simulink model "benchmark_ivan_PIANN"  (R2024b)
settings: Solver=FixedStepAuto  StartTime=0.0  StopTime=14  FixedStep=0.0001  RelTol=1e-5  AbsTol=1e-8  EnableMultiTasking=on
values from neighbouring files (symbols this model uses):
  b1 = csvread('./DAE_ANN/ANN/Biases/30_04_21/lstm_ann_pi_standard_fix_noSo4_rnn_1__100_16_b_3.csv')    [init_PI_ann.m]    (also in init_PI_ann_hier.m = csvread('./DAE_ANN/ANN/Biases/12_05_21/lstm_ann_pi_standard_; init_PI_ann_hier_v2.m = csvread('./DAE_ANN/ANN/Biases/12_05_21/lstm_ann_pi_standard_; init_PI_ann_lab.m = csvread('./DAE_ANN/ANN/Biases/12_05_21/lstm_ann_pi_standard_)
  b2 = csvread('./DAE_ANN/ANN/Biases/30_04_21/lstm_ann_pi_standard_fix_noSo4_rnn_1__100_16_b_3.csv')    [init_PI_ann.m]    (also in init_PI_ann_hier.m = csvread('./DAE_ANN/ANN/Biases/12_05_21/lstm_ann_pi_standard_; init_PI_ann_hier_v2.m = csvread('./DAE_ANN/ANN/Biases/12_05_21/lstm_ann_pi_standard_; init_PI_ann_lab.m = csvread('./DAE_ANN/ANN/Biases/12_05_21/lstm_ann_pi_standard_)
  b_last = csvread('./DAE_ANN/ANN/Biases/12_05_21/lstm_ann_pi_standard_fix_noSo4_last__100_1_b_2.csv')'    [init_PI_ann_hier.m]    (also in init_PI_ann_hier_v2.m; init_PI_ann_lab.m)
  b_out = csvread('./DAE_ANN/ANN/Biases/30_04_21/lstm_ann_pi_standard_fix_noSo4_final__100_16_b_3.csv')    [init_PI_ann.m]    (also in init_PI_ann_hier.m = csvread('./DAE_ANN/ANN/Biases/12_05_21/lstm_ann_pi_standard_; init_PI_ann_hier_v2.m = csvread('./DAE_ANN/ANN/Biases/12_05_21/lstm_ann_pi_standard_; init_PI_ann_lab.m = csvread('./DAE_ANN/ANN/Biases/12_05_21/lstm_ann_pi_standard_)
  ic_sw_Kla = 145*ones(n_sw,1)    [init_PI_ann.m]    (also in init_PI_ann_hier.m; init_PI_ann_hier_v2.m; init_PI_ann_lab.m)
  ic_sw_Snh4 = 6*ones(n_sw,1)    [init_PI_ann.m]    (also in init_PI_ann_hier.m; init_PI_ann_hier_v2.m; init_PI_ann_lab.m)
  ic_sw_Sno4 = 8*ones(n_sw,1)    [init_PI_ann.m]    (also in init_PI_ann_hier.m; init_PI_ann_hier_v2.m; init_PI_ann_lab.m)
  ic_sw_So4 = 3*ones(n_sw,1)    [init_PI_ann.m]    (also in init_PI_ann_hier.m; init_PI_ann_hier_v2.m; init_PI_ann_lab.m)
  ic_sw_So5 = 2*ones(n_sw,1)    [init_PI_ann.m]    (also in init_PI_ann_hier.m; init_PI_ann_hier_v2.m; init_PI_ann_lab.m)
  KLa5_max = 360    [sensorinit.m]
  max_Q4 = 100000    [sensorinit.m]
  max_SNH4 = 20    [sensorinit.m]
  max_SNO2 = 20    [sensorinit.m]
  max_SNO4 = 20    [sensorinit.m]
  max_SO4 = 10    [sensorinit.m]
  max_SO5 = 10    [sensorinit.m]    (also in setup_Prac5.m = 5)
  max_TSS4 = 10000    [sensorinit.m]
  mean_scaler_dir = csvread('./DAE_ANN/ANN/Scalers/30_04_21_lstm_ann_pi_standard_fix_noSo4/mean_scaler_lstm_ann_pi_standard_fix_noSo4.csv')    [init_PI_ann.m]    (also in init_PI_ann_hier.m = csvread('./DAE_ANN/ANN/Scalers/12_05_21_lstm_ann_pi_standard; init_PI_ann_hier_v2.m = csvread('./DAE_ANN/ANN/Scalers/12_05_21_lstm_ann_pi_standard; setup_Prac5.m = [(Q/k)^2, 1.9756, 0.0000, 0]')
  mean_scaler_dir_out = csvread('./DAE_ANN/ANN/Scalers/30_04_21_lstm_ann_pi_standard_fix_noSo4/mean_scaler_lstm_ann_pi_standard_fix_noSo4_out.csv')    [init_PI_ann.m]    (also in init_PI_ann_hier.m = csvread('./DAE_ANN/ANN/Scalers/12_05_21_lstm_ann_pi_standard; init_PI_ann_hier_v2.m = csvread('./DAE_ANN/ANN/Scalers/12_05_21_lstm_ann_pi_standard; setup_Prac5.m = 0)
  min_Q4 = 0    [sensorinit.m]
  min_SNH4 = 0    [sensorinit.m]
  min_SNO2 = 0    [sensorinit.m]
  min_SNO4 = 0    [sensorinit.m]
  min_SO5 = 0    [sensorinit.m]
  min_TSS4 = 0    [sensorinit.m]
  n_layers = 1    [init_PI_ann.m]    (also in init_PI_ann_hier.m; init_PI_ann_hier_v2.m; init_PI_ann_lab.m)
  n_sw = 16    [init_PI_ann.m]    (also in init_PI_ann_hier.m = 1; init_PI_ann_hier_v2.m = 1; init_PI_ann_lab.m = 1)
  n_sw_inverse = 16    [init_PI_ann.m]    (also in init_PI_ann_hier.m = 1; init_PI_ann_hier_v2.m = 1; init_PI_ann_lab.m = 1)
  noiseseed_Q4 = 1    [sensorinit.m]
  noiseseed_SNH4 = 2    [sensorinit.m]
  noiseseed_SNO2 = 2    [sensorinit.m]
  noiseseed_SNO4 = 2    [sensorinit.m]
  noiseseed_SO4 = 2    [sensorinit.m]
  noiseseed_SO5 = 1    [sensorinit.m]
  noiseseed_TSS4 = 1    [sensorinit.m]
  noisesource_Q4 = 1    [sensorinit.m]
  noisesource_SNH4 = 1    [sensorinit.m]
  noisesource_SNO2 = 1    [sensorinit.m]
  noisesource_SNO4 = 1    [sensorinit.m]
  noisesource_SO4 = 1    [sensorinit.m]
  noisesource_SO5 = 1    [sensorinit.m]
  noisesource_TSS4 = 1    [sensorinit.m]
  Qin0 = 18446    [states.mat]
  Qintr = 12141.8126939    [states.mat]
  Qintr_max = 5*Qin0    [sensorinit.m]
  Qintrawstate = 114243.527362    [states.mat]
  Qintrintstate = -116205.765277    [states.mat]
  SETTLERINIT = [12.5979803087 18.2981709885 29.6744598765 68.7829340492 352.293497132 353.981663079 351.499035887 351.323930185 355.679725774 6417.21684783 30 30 ... (80 elements, 1x80)]    [states.mat]
  Sno_mean = 1    [run_bsm1_PIANN_variable.m]
  SO5awstate = 469.399689831    [states.mat]
  SO5intstate = -450.70071346    [states.mat]
  SO5ref = 2    [run_bsm1_PIANN.m]    (also in run_bsm1_PIANN_variable.m)
  So_mean = 2    [run_bsm1_PIANN_variable.m]    (also in setup_Prac5.m = 0.2)
  std_Q4 = 0.025    [sensorinit.m]
  std_scaler_dir = csvread('./DAE_ANN/ANN/Scalers/30_04_21_lstm_ann_pi_standard_fix_noSo4/std_scaler_lstm_ann_pi_standard_fix_noSo4.csv')    [init_PI_ann.m]    (also in init_PI_ann_hier.m = csvread('./DAE_ANN/ANN/Scalers/12_05_21_lstm_ann_pi_standard; init_PI_ann_hier_v2.m = csvread('./DAE_ANN/ANN/Scalers/12_05_21_lstm_ann_pi_standard; setup_Prac5.m = [1, 0.7579, 0.05, 1]')
  std_scaler_dir_out = csvread('./DAE_ANN/ANN/Scalers/30_04_21_lstm_ann_pi_standard_fix_noSo4/std_scaler_lstm_ann_pi_standard_fix_noSo4_out.csv')    [init_PI_ann.m]    (also in init_PI_ann_hier.m = csvread('./DAE_ANN/ANN/Scalers/12_05_21_lstm_ann_pi_standard; init_PI_ann_hier_v2.m = csvread('./DAE_ANN/ANN/Scalers/12_05_21_lstm_ann_pi_standard; setup_Prac5.m = 1)
  std_SNH4 = 0.025    [sensorinit.m]
  std_SNO2 = 0.025    [sensorinit.m]
  std_SO4 = 0.025    [sensorinit.m]
  std_SO5 = 0.025    [sensorinit.m]
  std_TSS4 = 0.025    [sensorinit.m]
  T = 6.5201    [setup_Prac5.m]
  t_init = 7e-3    (= 0.007)    [run_bsm1.m]    (also in run_bsm1_PIANN_variable.m = 0.05)
  T_KLa5 = T90_KLa5/(24*60)/3.89    (= 0.000714081690945)    [sensorinit.m]
  T_Q4 = T90_Q4/(24*60)/3.89    (= 0.000178520422736)    [sensorinit.m]
  t_simulink = 1/96    (= 0.0104166666667)    [run_bsm1.m]    (also in run_bsm1_PIANN.m = -1; run_bsm1_PIANN_variable.m = 0; setup_Prac5.m = 0)
  T_SNH4 = T90_SNH4/(24*60)/11.7724    (= 0.000589891988417)    [sensorinit.m]
  T_SNO2 = T90_SNO2/(24*60)/11.7724    (= 0.000589891988417)    [sensorinit.m]
  T_SNO4 = T90_SNO4/(24*60)/11.7724    (= 0.000589891988417)    [sensorinit.m]
  T_SO5 = T90_SO5/(24*60)/3.89    (= 0.000178520422736)    [sensorinit.m]
  T_TSS4 = T90_TSS4/(24*60)/3.89    (= 0.000178520422736)    [sensorinit.m]
  t_zero_order = -1    [run_bsm1_PIANN.m]    (also in run_bsm1_PIANN_variable.m)
  u1 = csvread('./DAE_ANN/ANN/Weights/30_04_21/lstm_ann_pi_standard_fix_noSo4_rnn_1__100_16_U_3.csv')    [init_PI_ann.m]    (also in init_PI_ann_hier.m = csvread('./DAE_ANN/ANN/Weights/12_05_21/lstm_ann_pi_standard; init_PI_ann_hier_v2.m = csvread('./DAE_ANN/ANN/Weights/12_05_21/lstm_ann_pi_standard)
  u2 = csvread('./DAE_ANN/ANN/Weights/30_04_21/lstm_ann_pi_standard_fix_noSo4_rnn_1__100_16_U_3.csv')    [init_PI_ann.m]    (also in init_PI_ann_hier.m = csvread('./DAE_ANN/ANN/Weights/12_05_21/lstm_ann_pi_standard; init_PI_ann_hier_v2.m = csvread('./DAE_ANN/ANN/Weights/12_05_21/lstm_ann_pi_standard)
  useideal_KLa5 = 0    [run_bsm1.m]    (also in run_bsm1_PIANN.m = 1; run_bsm1_PIANN_variable.m = 1; sensorinit.m)
  useideal_Q4 = 1    [run_bsm1_PIANN.m]    (also in run_bsm1_PIANN_variable.m; sensorinit.m = 0)
  useideal_SNH4 = 0    [run_bsm1.m]    (also in run_bsm1_PIANN.m = 1; run_bsm1_PIANN_variable.m = 1; sensorinit.m)
  useideal_SNO2 = 1    [run_bsm1_PIANN.m]    (also in run_bsm1_PIANN_variable.m; sensorinit.m = 0)
  useideal_SNO4 = 0    [run_bsm1.m]    (also in run_bsm1_PIANN.m = 1; run_bsm1_PIANN_variable.m = 1; sensorinit.m)
  useideal_SO4 = 0    [run_bsm1.m]    (also in run_bsm1_PIANN.m = 1; run_bsm1_PIANN_variable.m = 1; sensorinit.m)
  useideal_SO5 = 0    [run_bsm1.m]    (also in run_bsm1_PIANN.m = 1; run_bsm1_PIANN_variable.m = 1; sensorinit.m)
  useideal_TSS4 = 1    [run_bsm1_PIANN.m]    (also in run_bsm1_PIANN_variable.m; sensorinit.m = 0)
  usenoise_Q4 = 0    [run_bsm1_PIANN.m]    (also in run_bsm1_PIANN_variable.m; sensorinit.m = 1)
  usenoise_SNH4 = 1    [run_bsm1.m]    (also in run_bsm1_PIANN.m = 0; run_bsm1_PIANN_variable.m = 0; sensorinit.m)
  usenoise_SNO2 = 0    [run_bsm1_PIANN.m]    (also in run_bsm1_PIANN_variable.m; sensorinit.m = 1)
  usenoise_SNO4 = 1    [run_bsm1.m]    (also in run_bsm1_PIANN.m = 0; run_bsm1_PIANN_variable.m = 0; sensorinit.m)
  usenoise_SO4 = 1    [run_bsm1.m]    (also in run_bsm1_PIANN.m = 0; run_bsm1_PIANN_variable.m = 0; sensorinit.m)
  usenoise_SO5 = 1    [run_bsm1.m]    (also in run_bsm1_PIANN.m = 0; run_bsm1_PIANN_variable.m = 0; sensorinit.m)
  usenoise_TSS4 = 0    [run_bsm1_PIANN.m]    (also in run_bsm1_PIANN_variable.m; sensorinit.m = 1)
  w1 = csvread('./DAE_ANN/ANN/Weights/30_04_21/lstm_ann_pi_standard_fix_noSo4_rnn_1__100_16_W_3.csv')    [init_PI_ann.m]    (also in init_PI_ann_hier.m = csvread('./DAE_ANN/ANN/Weights/12_05_21/lstm_ann_pi_standard; init_PI_ann_hier_v2.m = csvread('./DAE_ANN/ANN/Weights/12_05_21/lstm_ann_pi_standard; init_PI_ann_lab.m = csvread('./DAE_ANN/ANN/Weights/12_05_21/lstm_ann_pi_standard)
  w2 = csvread('./DAE_ANN/ANN/Weights/30_04_21/lstm_ann_pi_standard_fix_noSo4_rnn_1__100_16_W_3.csv')    [init_PI_ann.m]    (also in init_PI_ann_hier.m = csvread('./DAE_ANN/ANN/Weights/12_05_21/lstm_ann_pi_standard; init_PI_ann_hier_v2.m = csvread('./DAE_ANN/ANN/Weights/12_05_21/lstm_ann_pi_standard; init_PI_ann_lab.m = csvread('./DAE_ANN/ANN/Weights/12_05_21/lstm_ann_pi_standard)
  w_last = csvread('./DAE_ANN/ANN/Weights/12_05_21/lstm_ann_pi_standard_fix_noSo4_last__100_1_W_2.csv')    [init_PI_ann_hier.m]    (also in init_PI_ann_hier_v2.m; init_PI_ann_lab.m)
  w_out = csvread('./DAE_ANN/ANN/Weights/30_04_21/lstm_ann_pi_standard_fix_noSo4_final__100_16_W_3.csv')    [init_PI_ann.m]    (also in init_PI_ann_hier.m = csvread('./DAE_ANN/ANN/Weights/12_05_21/lstm_ann_pi_standard; init_PI_ann_hier_v2.m = csvread('./DAE_ANN/ANN/Weights/12_05_21/lstm_ann_pi_standard; init_PI_ann_lab.m = csvread('./DAE_ANN/ANN/Weights/12_05_21/lstm_ann_pi_standard)
  XINIT1 = [30 3.2250440682 1132.84750814 98.0848162551 2520.32093658 147.34360098 454.498440184 0.006943357113 3.54207658602 12.0720627837 1.35151294762 6.05742445882 ... (15 elements, 1x15)]    [states.mat]
  XINIT2 = [30 1.63865407136 1124.24951453 88.653599068 2501.35826654 146.001740625 452.094465666 5.17099136584e-05 1.14245691502 13.0383387996 0.796493225193 5.70045637375 ... (15 elements, 1x15)]    [states.mat]
  XINIT3 = [30 1.20592174915 1120.58961418 67.1871738861 2499.94635325 146.547839977 452.007772249 1.74081325353 6.26492922945 8.40116301472 0.827753486834 4.51387309735 ... (15 elements, 1x15)]    [states.mat]
  XINIT4 = [30 0.96656120797 1121.66055561 52.7833355811 2504.32671079 147.644975737 453.890499756 2.40137566232 11.073804945 3.99279026202 0.746788866766 3.70339113264 ... (15 elements, 1x15)]    [states.mat]
  XINIT5 = [30 0.803395489358 1124.12455116 43.2595495328 2508.23031357 148.499403125 456.322790044 2.11978031988 14.1356901459 1.15379834533 0.659650038761 3.15951382084 ... (15 elements, 1x15)]    [states.mat]
  XINITDELAY = [1466770.04249 1266021.87556 55799754.9774 5815431.95778 123179806.598 7263098.80912 22318785.5012 62039.7687555 416609.519268 588047.303413 143684.636473 343270.852984 ... (15 elements, 1x15)]    [states.mat]
undefined symbols (not defined in the file or in its folder): b_bottle, b_decoder_1, b_decoder_2, b_encoder_1, b_encoder_2, b_final, b_out_dae, carb1, carb2, carb3, carb4, carb5, DIM, Kfeedforward, KLa1, KLa2, KLa3, KLa4, KLa5offset, KQintr, KSO5, LAYER, magnitude, mean_scaler_dae, mean_scaler_dae_out, MODELTYPE, PAR1, PAR2, PAR3, PAR4, PAR5, Qffref, Qintroffset, QintrT, SETTLERPAR, SNO2ref, SOSAT1, SOSAT2, SOSAT3, SOSAT4, SOSAT5, std_scaler_dae, std_scaler_dae_out, TiQintr, TiSO5, TtQintr, TtSO5, u_decoder_1, u_decoder_2, u_encoder_1, u_encoder_2, useantiwindupQintr, useantiwindupSO5, VOL1, VOL2, VOL3, VOL4, VOL5, w_bottle, w_decoder_1 ... (+5)
libraries: dspindex x33
(part 4 of 4)

== matlab function benchmark_ivan_PIANN/SO5_control_paper/Filter_Prediction/DAE_lstm/DAE/Predict RNN ==
  data: data_in input; prediction output; w_encoder_1 parameter; u_encoder_1 parameter; b_encoder_1 parameter; w_encoder_2 parameter; u_encoder_2 parameter; b_encoder_2 parameter; w_decoder_1 parameter; u_decoder_1 parameter; b_decoder_1 parameter; w_decoder_2 parameter; u_decoder_2 parameter; b_decoder_2 parameter; w_out_dae parameter; b_out_dae parameter
function prediction   = predict_rnn(data_in, ...
    w_encoder_1, u_encoder_1, b_encoder_1, ...
    w_encoder_2, u_encoder_2, b_encoder_2, ...
    w_decoder_1, u_decoder_1, b_decoder_1, ...
    w_decoder_2, u_decoder_2, b_decoder_2, ...
    w_out_dae, b_out_dae)
%UNTITLED2 Summary of this function goes here
%   Detailed explanation goes here
    
    n_input = size(w_encoder_1,1);
    n_steps = 16;
    n_h_encoder_1 = size(u_encoder_1,1);
    n_h_encoder_2 = size(u_encoder_2,1);
    n_h_decoder_1 = n_h_encoder_2;
    n_h_decoder_2 = n_h_encoder_1;
    
%% Encoder 1

    w_i_1 = w_encoder_1(:,1:n_h_encoder_1);
    w_f_1 = w_encoder_1(:,n_h_encoder_1*1+1:n_h_encoder_1*2);
    w_C_1 = w_encoder_1(:,n_h_encoder_1*2+1:n_h_encoder_1*3);
    w_o_1 = w_encoder_1(:,n_h_encoder_1*3+1:end);

    u_i_1 = u_encoder_1(:,1:n_h_encoder_1);
    u_f_1 = u_encoder_1(:,n_h_encoder_1*1+1:n_h_encoder_1*2);
    u_C_1 = u_encoder_1(:,n_h_encoder_1*2+1:n_h_encoder_1*3);
    u_o_1 = u_encoder_1(:,n_h_encoder_1*3+1:end);
   
    b_i_1 = b_encoder_1(1:n_h_encoder_1)';
    b_f_1 = b_encoder_1(n_h_encoder_1*1+1:n_h_encoder_1*2)';
    b_C_1 = b_encoder_1(n_h_encoder_1*2+1:n_h_encoder_1*3)';
    b_o_1 = b_encoder_1(n_h_encoder_1*3+1:n_h_encoder_1*4)';


%% Encoder 2

    w_i_2 = w_encoder_2(:,1:n_h_encoder_2);
    w_f_2 = w_encoder_2(:,n_h_encoder_2*1+1:n_h_encoder_2*2);
    w_C_2 = w_encoder_2(:,n_h_encoder_2*2+1:n_h_encoder_2*3);
    w_o_2 = w_encoder_2(:,n_h_encoder_2*3+1:end);

    u_i_2 = u_encoder_2(:,1:n_h_encoder_2);
    u_f_2 = u_encoder_2(:,n_h_encoder_2*1+1:n_h_encoder_2*2);
    u_C_2 = u_encoder_2(:,n_h_encoder_2*2+1:n_h_encoder_2*3);
    u_o_2 = u_encoder_2(:,n_h_encoder_2*3+1:end);
    
    b_i_2 = b_encoder_2(1:n_h_encoder_2)';
    b_f_2 = b_encoder_2(n_h_encoder_2+1:n_h_encoder_2*2)';
    b_C_2 = b_encoder_2(n_h_encoder_2*2+1:n_h_encoder_2*3)';
    b_o_2 = b_encoder_2(n_h_encoder_2*3+1:n_h_encoder_2*4)';

%% Decoder 1

    w_i_3 = w_decoder_1(:,1:n_h_decoder_1);
    w_f_3 = w_decoder_1(:,n_h_decoder_1*1+1:n_h_decoder_1*2);
    w_C_3 = w_decoder_1(:,n_h_decoder_1*2+1:n_h_decoder_1*3);
    w_o_3 = w_decoder_1(:,n_h_decoder_1*3+1:end);

    u_i_3 = u_decoder_1(:,1:n_h_decoder_1);
    u_f_3 = u_decoder_1(:,n_h_decoder_1*1+1:n_h_decoder_1*2);
    u_C_3 = u_decoder_1(:,n_h_decoder_1*2+1:n_h_decoder_1*3);
    u_o_3 = u_decoder_1(:,n_h_decoder_1*3+1:end);
   
    b_i_3 = b_decoder_1(1:n_h_decoder_1)';
    b_f_3 = b_decoder_1(n_h_decoder_1*1+1:n_h_decoder_1*2)';
    b_C_3 = b_decoder_1(n_h_decoder_1*2+1:n_h_decoder_1*3)';
    b_o_3 = b_decoder_1(n_h_decoder_1*3+1:n_h_decoder_1*4)';


%% Decoder 2

    w_i_4 = w_decoder_2(:,1:n_h_decoder_2);
    w_f_4 = w_decoder_2(:,n_h_decoder_2*1+1:n_h_decoder_2*2);
    w_C_4 = w_decoder_2(:,n_h_decoder_2*2+1:n_h_decoder_2*3);
    w_o_4 = w_decoder_2(:,n_h_decoder_2*3+1:end);

    u_i_4 = u_decoder_2(:,1:n_h_decoder_2);
    u_f_4 = u_decoder_2(:,n_h_decoder_2*1+1:n_h_decoder_2*2);
    u_C_4 = u_decoder_2(:,n_h_decoder_2*2+1:n_h_decoder_2*3);
    u_o_4 = u_decoder_2(:,n_h_decoder_2*3+1:end);
    
    b_i_4 = b_decoder_2(1:n_h_decoder_2)';
    b_f_4 = b_decoder_2(n_h_decoder_2+1:n_h_decoder_2*2)';
    b_C_4 = b_decoder_2(n_h_decoder_2*2+1:n_h_decoder_2*3)';
    b_o_4 = b_decoder_2(n_h_decoder_2*3+1:n_h_decoder_2*4)';

%% Split data in four parts
                 
    j = 1;
        
    h_t1 = zeros(1, n_h_encoder_1);
    C_t1 = zeros(1, n_h_encoder_1);

    h_t2 = zeros(1, n_h_encoder_2);
    C_t2 = zeros(1, n_h_encoder_2);

    h_t3 = zeros(1, n_h_decoder_1);
    C_t3 = zeros(1, n_h_decoder_1);

    h_t4 = zeros(1, n_h_decoder_2);
    C_t4 = zeros(1, n_h_decoder_2);
    
    prediction = zeros(1,n_steps*n_input);
    prediction_aux = zeros(1,n_input);
    prediction_vect = zeros(1, n_steps*n_input);

    while j<=n_steps
        
        x_t = data_in(1+n_input*(j-1):n_input*j);
            
        f_t_1_nosig = ((x_t*w_f_1)+(h_t1*u_f_1)+(b_f_1));
        f_t_1 = 1./(1 + exp(-1.*(f_t_1_nosig)));
        i_t_1_nosig = ((x_t*w_i_1)+(h_t1*u_i_1)+b_i_1);
        i_t_1 = 1./(1 + exp(-1.*(i_t_1_nosig)));
        C_t1_new = tanh((x_t*w_C_1)+(h_t1*u_C_1)+b_C_1);
        C_t1 = (f_t_1).*C_t1 + i_t_1.*C_t1_new;
            
        o_t_1_nosig = ((x_t*w_o_1)+(h_t1*u_o_1)+b_o_1);
        o_t_1 = 1./(1 + exp(-1.*(o_t_1_nosig)));
        h_t1 = o_t_1.*tanh(C_t1);
        
        f_t_2_nosig = ((h_t1*w_f_2)+(h_t2*u_f_2)+(b_f_2));
        f_t_2 = 1./(1 + exp(-1.*(f_t_2_nosig)));
        i_t_2_nosig = ((h_t1*w_i_2)+(h_t2*u_i_2)+b_i_2);
        i_t_2 = 1./(1 + exp(-1.*(i_t_2_nosig)));
        C_t2_new = tanh((h_t1*w_C_2)+(h_t2*u_C_2)+b_C_2);
        C_t2 = (f_t_2).*C_t2 + i_t_2.*C_t2_new;
            
        o_t_2_nosig = ((h_t1*w_o_2)+(h_t2*u_o_2)+b_o_2);
        o_t_2 = 1./(1 + exp(-1.*(o_t_2_nosig)));
        h_t2 = o_t_2.*tanh(C_t2);
            
        j = j+1;
    end
    
    h_t2_aux = repmat(h_t2, n_steps,1);
    
    j = 1;
    while j<=n_steps
        
        h_t2_after = h_t2_aux(j,:);
        
        f_t_3_nosig = ((h_t2_after*w_f_3)+(h_t3*u_f_3)+(b_f_3));
        f_t_3 = 1./(1 + exp(-1.*(f_t_3_nosig)));
        i_t_3_nosig = ((h_t2_after*w_i_3)+(h_t3*u_i_3)+b_i_3);
        i_t_3 = 1./(1 + exp(-1.*(i_t_3_nosig)));
        C_t3_new = tanh((h_t2_after*w_C_3)+(h_t3*u_C_3)+b_C_3);
        C_t3 = (f_t_3).*C_t3 + i_t_3.*C_t3_new;
            
        o_t_3_nosig = ((h_t2_after*w_o_3)+(h_t3*u_o_3)+b_o_3);
        o_t_3 = 1./(1 + exp(-1.*(o_t_3_nosig)));
        h_t3 = o_t_3.*tanh(C_t3);
        
        
        f_t_4_nosig = ((h_t3*w_f_4)+(h_t4*u_f_4)+(b_f_4));
        f_t_4 = 1./(1 + exp(-1.*(f_t_4_nosig)));
        i_t_4_nosig = ((h_t3*w_i_4)+(h_t4*u_i_4)+b_i_4);
        i_t_4 = 1./(1 + exp(-1.*(i_t_4_nosig)));
        C_t4_new = tanh((h_t3*w_C_4)+(h_t4*u_C_4)+b_C_4);
        C_t4 = (f_t_4).*C_t4 + i_t_4.*C_t4_new;
            
        o_t_4_nosig = ((h_t3*w_o_4)+(h_t4*u_o_4)+b_o_4);
        o_t_4 = 1./(1 + exp(-1.*(o_t_4_nosig)));
        h_t4 = o_t_4.*tanh(C_t4);
        
        prediction_aux = h_t4*w_out_dae + b_out_dae';
        
        prediction_vect(1+4*(j-1):4*j)=prediction_aux;               
        j = j+1;
    end
    prediction = prediction_vect;
end

== matlab function benchmark_ivan_PIANN/SO5_control_paper/Filter_Prediction/DAE_lstm/Data Preprocesing Direct/Normalizer1/Normalization Values ==
  data: mean_scaler_dae parameter; data_norm output; std_scaler_dae parameter; data_input input
function data_norm = scaler(mean_scaler_dae, std_scaler_dae, data_input)
%#codegen

mean_output_dae = repmat(mean_scaler_dae',[16,1]);
std_output_dae = repmat(std_scaler_dae', [16,1]);

data_norm = (data_input - mean_output_dae)./std_output_dae;

== matlab function benchmark_ivan_PIANN/SO5_control_paper/Filter_Prediction/DAE_lstm/Data Preprocessing Direct1/Denormalization Values ==
  data: mean_scaler_dae_out parameter; data_dir output; std_scaler_dae_out parameter; data_input input
function data_dir = descaler(mean_scaler_dae_out, std_scaler_dae_out, data_input)
%#codegen
data_dir = zeros(1, 64);

mean_output_3 = repmat(mean_scaler_dae_out',1,16);
std_output_3 = repmat(std_scaler_dae_out', 1,16);

data_dir = std_output_3.*data_input + mean_output_3;

== matlab function benchmark_ivan_PIANN/SO5_control_paper/Filter_Prediction/DAE_lstm/MATLAB Function ==
  data: data_in input; data_out output
function data_out = reshape_out_dae(data_in)
    
    data_in_aux = zeros(length(data_in),1);
    data_out_aux = zeros(3,16);
    data_out = zeros(16, 3);
    
    data_in_aux = data_in';
    data_out_aux = reshape(data_in_aux, 3, 16);
    
data_out = data_out_aux';

== matlab function benchmark_ivan_PIANN/SO5_control_paper/Filter_Prediction/Direct Prediction LSTM4/Data Preprocesing Direct/Normalization Values ==
  data: mean_scaler_dir parameter; data_norm output; std_scaler_dir parameter; data_input input
function data_norm = scaler(mean_scaler_dir, std_scaler_dir, data_input)
%#codegen
mean_output_2 = repmat(mean_scaler_dir',[16,1]);
std_output_2 = repmat(std_scaler_dir', [16,1]);

data_norm = (data_input - mean_output_2)./std_output_2;

== matlab function benchmark_ivan_PIANN/SO5_control_paper/Filter_Prediction/Direct Prediction LSTM4/Data Preprocessing Direct1/Denormalization Values ==
  data: mean_scaler_dir_out parameter; data_dir output; std_scaler_dir_out parameter; data_input input
function data_dir = descaler(mean_scaler_dir_out, std_scaler_dir_out, data_input)
%#codegen

mean_output_2 = mean_scaler_dir_out;
std_output_2 = std_scaler_dir_out;

data_dir = std_output_2.*data_input + mean_output_2;

== matlab function benchmark_ivan_PIANN/SO5_control_paper/Filter_Prediction/Direct Prediction LSTM4/Direct ANN/Predict RNN Ntot Keras ==
  data: data_in input; prediction output; w1 parameter; u1 parameter; w2 parameter; u2 parameter; w_out parameter; b1 parameter; b2 parameter; b_out parameter; n_layers parameter; n_sw parameter
function prediction = predict_rnn(data_in, w1, u1, w2, u2, w_out, b1, b2, b_out, n_layers, n_sw)
%#codegen
    
    prediction = 0;

    dim_w1 = size(w1);
    dim_w2 = size(w2);
    n_input = dim_w1(1);
    n_steps = n_sw;
    n_hidden = dim_w1(2)/4;
    
    %% Layer 1

    w_i_1 = w1(:,1:n_hidden);
    w_f_1 = w1(:,n_hidden*1+1:n_hidden*2);
    w_C_1 = w1(:,n_hidden*2+1:n_hidden*3);
    w_o_1 = w1(:,n_hidden*3+1:end);

    u_i_1 = u1(:,1:n_hidden);
    u_f_1 = u1(:,n_hidden*1+1:n_hidden*2);
    u_C_1 = u1(:,n_hidden*2+1:n_hidden*3);
    u_o_1 = u1(:,n_hidden*3+1:end);
   
    b_i_1 = b1(1:n_hidden)';
    b_f_1 = b1(n_hidden*1+1:n_hidden*2)';
    b_C_1 = b1(n_hidden*2+1:n_hidden*3)';
    b_o_1 = b1(n_hidden*3+1:n_hidden*4)';

%% Layer 2

    w_i_2 = w2(:,1:n_hidden);
    w_f_2 = w2(:,n_hidden*1+1:n_hidden*2);
    w_C_2 = w2(:,n_hidden*2+1:n_hidden*3);
    w_o_2 = w2(:,n_hidden*3+1:end);

    u_i_2 = u2(:,1:n_hidden);
    u_f_2 = u2(:,n_hidden*1+1:n_hidden*2);
    u_C_2 = u2(:,n_hidden*2+1:n_hidden*3);
    u_o_2 = u2(:,n_hidden*3+1:end);
    
    b_i_2 = b2(1:n_hidden)';
    b_f_2 = b2(n_hidden+1:n_hidden*2)';
    b_C_2 = b2(n_hidden*2+1:n_hidden*3)';
    b_o_2 = b2(n_hidden*3+1:n_hidden*4)';

%% Split data in four parts
                 
    j = 1;
        
    h_t1 = zeros(1, n_hidden);
    C_t1 = zeros(1, n_hidden);

    h_t2 = zeros(1, n_hidden);
    C_t2 = zeros(1, n_hidden);
    
    prediction_aux = 0;
    
    while j<=n_steps
        
        x_t = data_in(1+n_input*(j-1):n_input*j);
            
        f_t_1_nosig = ((x_t*w_f_1)+(h_t1*u_f_1)+(b_f_1));
        f_t_1 = 1./(1 + exp(-1.*(f_t_1_nosig)));
        i_t_1_nosig = ((x_t*w_i_1)+(h_t1*u_i_1)+b_i_1);
        i_t_1 = 1./(1 + exp(-1.*(i_t_1_nosig)));
        C_t1_new = tanh((x_t*w_C_1)+(h_t1*u_C_1)+b_C_1);
        C_t1 = (f_t_1).*C_t1 + i_t_1.*C_t1_new;
            
        o_t_1_nosig = ((x_t*w_o_1)+(h_t1*u_o_1)+b_o_1);
        o_t_1 = 1./(1 + exp(-1.*(o_t_1_nosig)));
        h_t1 = o_t_1.*tanh(C_t1);
        
%         f_t_2_nosig = ((h_t1*w_f_2)+(h_t2*u_f_2)+(b_f_2+1));
%         f_t_2 = 1./(1 + exp(-1.*(f_t_2_nosig)));
%         i_t_2_nosig = ((h_t1*w_i_2)+(h_t2*u_i_2)+b_i_2);
%         i_t_2 = 1./(1 + exp(-1.*(i_t_2_nosig)));
%         C_t2_new = tanh((h_t1*w_C_2)+(h_t2*u_C_2)+b_C_2);
%         C_t2 = f_t_2.*C_t2 + i_t_2.*C_t2_new;
% 
%         o_t_2_nosig = ((h_t1*w_o_2)+(h_t2*u_o_2)+b_o_2);
%         o_t_2 = 1./(1 + exp(-1.*(o_t_2_nosig)));
%         h_t2 = o_t_2.*tanh(C_t2);    

        prediction_aux = h_t1*w_out + b_out;
                        
        j = j+1;
    end
    prediction = prediction_aux;
end

== matlab function benchmark_ivan_PIANN/SO5_control_paper/Filter_Prediction/DAE_MLP3/DAE/Predict RNN ==
  data: data_in input; prediction output; w_encoder_1 parameter; b_encoder_1 parameter; w_encoder_2 parameter; b_encoder_2 parameter; w_bottle parameter; b_bottle parameter; w_decoder_1 parameter; b_decoder_1 parameter; w_decoder_2 parameter; b_decoder_2 parameter; w_final parameter; b_final parameter
function prediction = predict_rnn(data_in, w_encoder_1, b_encoder_1, ...
    w_encoder_2, b_encoder_2, ...
    w_bottle, b_bottle, ...
    w_decoder_1, b_decoder_1, ...
    w_decoder_2, b_decoder_2, ...
    w_final, b_final)
%#codegen
    
    prediction = zeros(1,64);

    enc_1 = data_in*w_encoder_1 + b_encoder_1;
    enc_1(enc_1<0) = 0;
    enc_1_relu = enc_1;
    
    enc_2 = enc_1_relu*w_encoder_2 + b_encoder_2;
    enc_2(enc_2<0) = 0;
    enc_2_relu = enc_2;
    
    bottle = enc_2_relu*w_bottle + b_bottle;
    bottle(bottle<0) = 0;
    bottle_relu = bottle;
    
    dec_1 = bottle_relu*w_decoder_1 + b_decoder_1;
    dec_1(dec_1<0) = 0;
    dec_1_relu = dec_1;

    dec_2 = dec_1_relu*w_decoder_2 + b_decoder_2;
    dec_2(dec_2<0) = 0;
    dec_2_relu = dec_2;
    
    prediction = dec_2_relu*w_final + b_final;
end

== matlab function benchmark_ivan_PIANN/SO5_control_paper/Filter_Prediction/DAE_MLP3/Data Preprocesing Direct/Normalization Values ==
  data: mean_scaler_dae parameter; data_norm output; std_scaler_dae parameter; data_input input
function data_norm = scaler(mean_scaler_dae, std_scaler_dae, data_input)
%#codegen

mean_output_dae = mean_scaler_dae';
std_output_dae = std_scaler_dae';

data_norm = (data_input - mean_output_dae)./std_output_dae;

== matlab function benchmark_ivan_PIANN/SO5_control_paper/Filter_Prediction/DAE_MLP3/Data Preprocessing Direct1/Denormalization Values ==
  data: mean_scaler_dae_out parameter; data_dir output; std_scaler_dae_out parameter; data_input input
function data_dir = descaler(mean_scaler_dae_out, std_scaler_dae_out, data_input)
%#codegen
data_dir = zeros(1, 64);

mean_output_3 = mean_scaler_dae_out';
std_output_3 = std_scaler_dae_out';

data_dir = std_output_3.*data_input + mean_output_3;

== matlab function benchmark_ivan_PIANN/Direct Prediction 2 LSTM SO1/Data Preprocessing Direct1/Denormalization Values ==
  data: mean_scaler_dir_out parameter; data_dir output; std_scaler_dir_out parameter; data_input input
function data_dir = descaler(mean_scaler_dir_out, std_scaler_dir_out, data_input)
%#codegen

mean_output_2 = mean_scaler_dir_out;
std_output_2 = std_scaler_dir_out;

data_dir = std_output_2.*data_input + mean_output_2;

== matlab function benchmark_ivan_PIANN/Direct Prediction 2 LSTM SO1/Direct ANN1/Predict RNN Ntot Keras ==
  data: data_in input; prediction output; w1 parameter; u1 parameter; w2 parameter; u2 parameter; b1 parameter; b2 parameter; w_out parameter; b_out parameter; n_layers parameter; n_sw parameter; w_last parameter; b_last parameter
function prediction = predict_rnn(data_in, w1, u1, w2, u2, b1, b2, w_out, b_out, n_layers, n_sw, w_last, b_last)
%#codegen
    
    prediction = 0;

    dim_w1 = size(w1);
    dim_w2 = size(w2);
    n_input = dim_w1(1);
    n_steps = n_sw;
    n_hidden = dim_w1(2)/4;
    n_hidden_2 = 50;
    
    %% Layer 1

    w_i_1 = w1(:,1:n_hidden);
    w_f_1 = w1(:,n_hidden*1+1:n_hidden*2);
    w_C_1 = w1(:,n_hidden*2+1:n_hidden*3);
    w_o_1 = w1(:,n_hidden*3+1:end);

    u_i_1 = u1(:,1:n_hidden);
    u_f_1 = u1(:,n_hidden*1+1:n_hidden*2);
    u_C_1 = u1(:,n_hidden*2+1:n_hidden*3);
    u_o_1 = u1(:,n_hidden*3+1:end);
   
    b_i_1 = b1(1:n_hidden)';
    b_f_1 = b1(n_hidden*1+1:n_hidden*2)';
    b_C_1 = b1(n_hidden*2+1:n_hidden*3)';
    b_o_1 = b1(n_hidden*3+1:n_hidden*4)';

%% Layer 2

    w_i_2 = w2(:,1:n_hidden_2);
    w_f_2 = w2(:,n_hidden_2*1+1:n_hidden_2*2);
    w_C_2 = w2(:,n_hidden_2*2+1:n_hidden_2*3);
    w_o_2 = w2(:,n_hidden_2*3+1:end);

    u_i_2 = u2(:,1:n_hidden_2);
    u_f_2 = u2(:,n_hidden_2*1+1:n_hidden_2*2);
    u_C_2 = u2(:,n_hidden_2*2+1:n_hidden_2*3);
    u_o_2 = u2(:,n_hidden_2*3+1:end);
    
    b_i_2 = b2(1:n_hidden_2)';
    b_f_2 = b2(n_hidden_2+1:n_hidden_2*2)';
    b_C_2 = b2(n_hidden_2*2+1:n_hidden_2*3)';
    b_o_2 = b2(n_hidden_2*3+1:n_hidden_2*4)';

%% Split data in four parts
                 
    j = 1;
        
    h_t1 = zeros(1, n_hidden);
    C_t1 = zeros(1, n_hidden);

    h_t2 = zeros(1, n_hidden_2);
    C_t2 = zeros(1, n_hidden_2);
    
    prediction_aux = 0;
    
    while j<=n_steps
        
        x_t = data_in(1+n_input*(j-1):n_input*j);
            
        f_t_1_nosig = ((x_t*w_f_1)+(h_t1*u_f_1)+(b_f_1));
        f_t_1 = 1./(1 + exp(-1.*(f_t_1_nosig)));
        i_t_1_nosig = ((x_t*w_i_1)+(h_t1*u_i_1)+b_i_1);
        i_t_1 = 1./(1 + exp(-1.*(i_t_1_nosig)));
        C_t1_new = tanh((x_t*w_C_1)+(h_t1*u_C_1)+b_C_1);
        C_t1 = (f_t_1).*C_t1 + i_t_1.*C_t1_new;
            
        o_t_1_nosig = ((x_t*w_o_1)+(h_t1*u_o_1)+b_o_1);
        o_t_1 = 1./(1 + exp(-1.*(o_t_1_nosig)));
        h_t1 = o_t_1.*tanh(C_t1);
        
        f_t_2_nosig = ((h_t1*w_f_2)+(h_t2*u_f_2)+(b_f_2+1));
        f_t_2 = 1./(1 + exp(-1.*(f_t_2_nosig)));
        i_t_2_nosig = ((h_t1*w_i_2)+(h_t2*u_i_2)+b_i_2);
        i_t_2 = 1./(1 + exp(-1.*(i_t_2_nosig)));
        C_t2_new = tanh((h_t1*w_C_2)+(h_t2*u_C_2)+b_C_2);
        C_t2 = f_t_2.*C_t2 + i_t_2.*C_t2_new;

        o_t_2_nosig = ((h_t1*w_o_2)+(h_t2*u_o_2)+b_o_2);
        o_t_2 = 1./(1 + exp(-1.*(o_t_2_nosig)));
        h_t2 = o_t_2.*tanh(C_t2);    

        prediction_aux_2 = h_t2*w_last + b_last;
        
        prediction_aux_2(prediction_aux_2<0) = 0;
        
        prediction_aux = prediction_aux_2*w_out + b_out;

                        
        j = j+1;
    end
    prediction = prediction_aux;
end

== matlab function benchmark_ivan_PIANN/Direct Prediction LSTM3/Data Preprocesing Direct/Normalizer1/Normalization Values ==
  data: mean_scaler_dir parameter; data_norm output; std_scaler_dir parameter; data_input input
function data_norm = scaler(mean_scaler_dir, std_scaler_dir, data_input)
%#codegen

mean_output_2 = repmat(mean_scaler_dir',[16,1]);
std_output_2 = repmat(std_scaler_dir', [16,1]);

data_norm = (data_input - mean_output_2)./std_output_2;

== matlab function benchmark_ivan_PIANN/Direct Prediction 2 LSTM SO1/Data Preprocesing Direct/Normalizer1/Normalization Values ==
  data: mean_scaler_dir parameter; data_norm output; std_scaler_dir parameter; data_input input
function data_norm = scaler(mean_scaler_dir, std_scaler_dir, data_input)
%#codegen

mean_output_2 = mean_scaler_dir';
std_output_2 = std_scaler_dir';

data_norm = (data_input - mean_output_2)./std_output_2;

== matlab function benchmark_ivan_PIANN/Direct Prediction LSTM3/Data Preprocessing Direct1/Denormalization Values ==
  data: mean_scaler_dir_out parameter; data_dir output; std_scaler_dir_out parameter; data_input input
function data_dir = descaler(mean_scaler_dir_out, std_scaler_dir_out, data_input)
%#codegen

mean_output_2 = mean_scaler_dir_out;
std_output_2 = std_scaler_dir_out;

data_dir = std_output_2.*data_input + mean_output_2;

== matlab function benchmark_ivan_PIANN/Direct Prediction LSTM3/Direct ANN/Predict RNN Ntot Keras ==
  data: data_in input; prediction output; w1 parameter; u1 parameter; w2 parameter; u2 parameter; w_out parameter; b1 parameter; b2 parameter; b_out parameter; n_layers parameter; n_sw parameter
function prediction = predict_rnn(data_in, w1, u1, w2, u2, w_out, b1, b2, b_out, n_layers, n_sw)
%#codegen
    
    prediction = 0;

    dim_w1 = size(w1);
    dim_w2 = size(w2);
    n_input = dim_w1(1);
    n_steps = n_sw;
    n_hidden = dim_w1(2)/4;
    
    %% Layer 1

    w_i_1 = w1(:,1:n_hidden);
    w_f_1 = w1(:,n_hidden*1+1:n_hidden*2);
    w_C_1 = w1(:,n_hidden*2+1:n_hidden*3);
    w_o_1 = w1(:,n_hidden*3+1:end);

    u_i_1 = u1(:,1:n_hidden);
    u_f_1 = u1(:,n_hidden*1+1:n_hidden*2);
    u_C_1 = u1(:,n_hidden*2+1:n_hidden*3);
    u_o_1 = u1(:,n_hidden*3+1:end);
   
    b_i_1 = b1(1:n_hidden)';
    b_f_1 = b1(n_hidden*1+1:n_hidden*2)';
    b_C_1 = b1(n_hidden*2+1:n_hidden*3)';
    b_o_1 = b1(n_hidden*3+1:n_hidden*4)';

%% Layer 2

    w_i_2 = w2(:,1:n_hidden);
    w_f_2 = w2(:,n_hidden*1+1:n_hidden*2);
    w_C_2 = w2(:,n_hidden*2+1:n_hidden*3);
    w_o_2 = w2(:,n_hidden*3+1:end);

    u_i_2 = u2(:,1:n_hidden);
    u_f_2 = u2(:,n_hidden*1+1:n_hidden*2);
    u_C_2 = u2(:,n_hidden*2+1:n_hidden*3);
    u_o_2 = u2(:,n_hidden*3+1:end);
    
    b_i_2 = b2(1:n_hidden)';
    b_f_2 = b2(n_hidden+1:n_hidden*2)';
    b_C_2 = b2(n_hidden*2+1:n_hidden*3)';
    b_o_2 = b2(n_hidden*3+1:n_hidden*4)';

%% Split data in four parts
                 
    j = 1;
        
    h_t1 = zeros(1, n_hidden);
    C_t1 = zeros(1, n_hidden);

    h_t2 = zeros(1, n_hidden);
    C_t2 = zeros(1, n_hidden);
    
    prediction_aux = 0;
    
    while j<=n_steps
        
        x_t = data_in(1+n_input*(j-1):n_input*j);
            
        f_t_1_nosig = ((x_t*w_f_1)+(h_t1*u_f_1)+(b_f_1));
        f_t_1 = 1./(1 + exp(-1.*(f_t_1_nosig)));
        i_t_1_nosig = ((x_t*w_i_1)+(h_t1*u_i_1)+b_i_1);
        i_t_1 = 1./(1 + exp(-1.*(i_t_1_nosig)));
        C_t1_new = tanh((x_t*w_C_1)+(h_t1*u_C_1)+b_C_1);
        C_t1 = (f_t_1).*C_t1 + i_t_1.*C_t1_new;
            
        o_t_1_nosig = ((x_t*w_o_1)+(h_t1*u_o_1)+b_o_1);
        o_t_1 = 1./(1 + exp(-1.*(o_t_1_nosig)));
        h_t1 = o_t_1.*tanh(C_t1);
        
%         f_t_2_nosig = ((h_t1*w_f_2)+(h_t2*u_f_2)+(b_f_2+1));
%         f_t_2 = 1./(1 + exp(-1.*(f_t_2_nosig)));
%         i_t_2_nosig = ((h_t1*w_i_2)+(h_t2*u_i_2)+b_i_2);
%         i_t_2 = 1./(1 + exp(-1.*(i_t_2_nosig)));
%         C_t2_new = tanh((h_t1*w_C_2)+(h_t2*u_C_2)+b_C_2);
%         C_t2 = f_t_2.*C_t2 + i_t_2.*C_t2_new;
% 
%         o_t_2_nosig = ((h_t1*w_o_2)+(h_t2*u_o_2)+b_o_2);
%         o_t_2 = 1./(1 + exp(-1.*(o_t_2_nosig)));
%         h_t2 = o_t_2.*tanh(C_t2);    

        prediction_aux = h_t1*w_out + b_out;
                        
        j = j+1;
    end
    prediction = prediction_aux;
end

== matlab function benchmark_ivan_PIANN/SO5_control1/Filter_Prediction1/DAE_MLP2/Predict RNN ==
  data: data_in input; prediction output; w_encoder_1 parameter; b_encoder_1 parameter; w_encoder_2 parameter; b_encoder_2 parameter; w_bottle parameter; b_bottle parameter; w_decoder_1 parameter; b_decoder_1 parameter; w_decoder_2 parameter; b_decoder_2 parameter; w_final parameter; b_final parameter
function prediction = predict_rnn(data_in, w_encoder_1, b_encoder_1, ...
    w_encoder_2, b_encoder_2, ...
    w_bottle, b_bottle, ...
    w_decoder_1, b_decoder_1, ...
    w_decoder_2, b_decoder_2, ...
    w_final, b_final)
%#codegen
    
    prediction = zeros(1,48);

    enc_1 = data_in*w_encoder_1 + b_encoder_1;
    enc_1(enc_1<0) = 0;
    enc_1_relu = enc_1;
    
    enc_2 = enc_1_relu*w_encoder_2 + b_encoder_2;
    enc_2(enc_2<0) = 0;
    enc_2_relu = enc_2;
    
    bottle = enc_2_relu*w_bottle + b_bottle;
    bottle(bottle<0) = 0;
    bottle_relu = bottle;
    
    dec_1 = bottle_relu*w_decoder_1 + b_decoder_1;
    dec_1(dec_1<0) = 0;
    dec_1_relu = dec_1;

    dec_2 = dec_1_relu*w_decoder_2 + b_decoder_2;
    dec_2(dec_2<0) = 0;
    dec_2_relu = dec_2;
    
    prediction = dec_2_relu*w_final + b_final;
end

== matlab function benchmark_ivan_PIANN/SO5_control1/Filter_Prediction1/Direct Prediction LSTM4/Normalization Values ==
  data: mean_scaler_dir parameter; data_norm output; std_scaler_dir parameter; data_input input
function data_norm = scaler(mean_scaler_dir, std_scaler_dir, data_input)
%#codegen

mean_output_2 = repmat(mean_scaler_dir',[16,1]);
std_output_2 = repmat(std_scaler_dir', [16,1]);

data_norm = (data_input - mean_output_2)./std_output_2;

== matlab function benchmark_ivan_PIANN/SO5_control1/Filter_Prediction1/Direct Prediction LSTM4/Predict RNN Ntot Keras ==
  data: data_in input; prediction output; w1 parameter; u1 parameter; w2 parameter; u2 parameter; w_out parameter; b1 parameter; b2 parameter; b_out parameter; n_layers parameter; n_sw parameter
function prediction = predict_rnn(data_in, w1, u1, w2, u2, w_out, b1, b2, b_out, n_layers, n_sw)
%#codegen
    
    prediction = 0;

    dim_w1 = size(w1);
    dim_w2 = size(w2);
    n_input = dim_w1(1);
    n_steps = n_sw;
    n_hidden = dim_w1(2)/4;
    
    %% Layer 1

    w_i_1 = w1(:,1:n_hidden);
    w_f_1 = w1(:,n_hidden*1+1:n_hidden*2);
    w_C_1 = w1(:,n_hidden*2+1:n_hidden*3);
    w_o_1 = w1(:,n_hidden*3+1:end);

    u_i_1 = u1(:,1:n_hidden);
    u_f_1 = u1(:,n_hidden*1+1:n_hidden*2);
    u_C_1 = u1(:,n_hidden*2+1:n_hidden*3);
    u_o_1 = u1(:,n_hidden*3+1:end);
   
    b_i_1 = b1(1:n_hidden)';
    b_f_1 = b1(n_hidden*1+1:n_hidden*2)';
    b_C_1 = b1(n_hidden*2+1:n_hidden*3)';
    b_o_1 = b1(n_hidden*3+1:n_hidden*4)';

%% Layer 2

    w_i_2 = w2(:,1:n_hidden);
    w_f_2 = w2(:,n_hidden*1+1:n_hidden*2);
    w_C_2 = w2(:,n_hidden*2+1:n_hidden*3);
    w_o_2 = w2(:,n_hidden*3+1:end);

    u_i_2 = u2(:,1:n_hidden);
    u_f_2 = u2(:,n_hidden*1+1:n_hidden*2);
    u_C_2 = u2(:,n_hidden*2+1:n_hidden*3);
    u_o_2 = u2(:,n_hidden*3+1:end);
    
    b_i_2 = b2(1:n_hidden)';
    b_f_2 = b2(n_hidden+1:n_hidden*2)';
    b_C_2 = b2(n_hidden*2+1:n_hidden*3)';
    b_o_2 = b2(n_hidden*3+1:n_hidden*4)';

%% Split data in four parts
                 
    j = 1;
        
    h_t1 = zeros(1, n_hidden);
    C_t1 = zeros(1, n_hidden);

    h_t2 = zeros(1, n_hidden);
    C_t2 = zeros(1, n_hidden);
    
    prediction_aux = 0;
    
    while j<=n_steps
        
        x_t = data_in(1+n_input*(j-1):n_input*j);
            
        f_t_1_nosig = ((x_t*w_f_1)+(h_t1*u_f_1)+(b_f_1));
        f_t_1 = 1./(1 + exp(-1.*(f_t_1_nosig)));
        i_t_1_nosig = ((x_t*w_i_1)+(h_t1*u_i_1)+b_i_1);
        i_t_1 = 1./(1 + exp(-1.*(i_t_1_nosig)));
        C_t1_new = tanh((x_t*w_C_1)+(h_t1*u_C_1)+b_C_1);
        C_t1 = (f_t_1).*C_t1 + i_t_1.*C_t1_new;
            
        o_t_1_nosig = ((x_t*w_o_1)+(h_t1*u_o_1)+b_o_1);
        o_t_1 = 1./(1 + exp(-1.*(o_t_1_nosig)));
        h_t1 = o_t_1.*tanh(C_t1);
        
%         f_t_2_nosig = ((h_t1*w_f_2)+(h_t2*u_f_2)+(b_f_2+1));
%         f_t_2 = 1./(1 + exp(-1.*(f_t_2_nosig)));
%         i_t_2_nosig = ((h_t1*w_i_2)+(h_t2*u_i_2)+b_i_2);
%         i_t_2 = 1./(1 + exp(-1.*(i_t_2_nosig)));
%         C_t2_new = tanh((h_t1*w_C_2)+(h_t2*u_C_2)+b_C_2);
%         C_t2 = f_t_2.*C_t2 + i_t_2.*C_t2_new;
% 
%         o_t_2_nosig = ((h_t1*w_o_2)+(h_t2*u_o_2)+b_o_2);
%         o_t_2 = 1./(1 + exp(-1.*(o_t_2_nosig)));
%         h_t2 = o_t_2.*tanh(C_t2);    

        prediction_aux = h_t1*w_out + b_out;
                        
        j = j+1;
    end
    prediction = prediction_aux;
end

== matlab function benchmark_ivan_PIANN/SO5_control_paper/Filter_Prediction/DAE_MLP1/DAE/Predict RNN ==
  data: data_in input; prediction output; w_encoder_1 parameter; b_encoder_1 parameter; w_encoder_2 parameter; b_encoder_2 parameter; w_bottle parameter; b_bottle parameter; w_decoder_1 parameter; b_decoder_1 parameter; w_decoder_2 parameter; b_decoder_2 parameter; w_final parameter; b_final parameter
function prediction = predict_rnn(data_in, w_encoder_1, b_encoder_1, ...
    w_encoder_2, b_encoder_2, ...
    w_bottle, b_bottle, ...
    w_decoder_1, b_decoder_1, ...
    w_decoder_2, b_decoder_2, ...
    w_final, b_final)
%#codegen
    
    prediction = zeros(1,48);

    enc_1 = data_in*w_encoder_1 + b_encoder_1;
    enc_1(enc_1<0) = 0;
    enc_1_relu = enc_1;
    
    enc_2 = enc_1_relu*w_encoder_2 + b_encoder_2;
    enc_2(enc_2<0) = 0;
    enc_2_relu = enc_2;
    
    bottle = enc_2_relu*w_bottle + b_bottle;
    bottle(bottle<0) = 0;
    bottle_relu = bottle;
    
    dec_1 = bottle_relu*w_decoder_1 + b_decoder_1;
    dec_1(dec_1<0) = 0;
    dec_1_relu = dec_1;

    dec_2 = dec_1_relu*w_decoder_2 + b_decoder_2;
    dec_2(dec_2<0) = 0;
    dec_2_relu = dec_2;
    
    prediction = dec_2_relu*w_final + b_final;
end

== matlab function benchmark_ivan_PIANN/SO5_control_paper/Filter_Prediction/DAE_MLP1/Data Preprocesing Direct/Normalization Values ==
  data: mean_scaler_dae parameter; data_norm output; std_scaler_dae parameter; data_input input
function data_norm = scaler(mean_scaler_dae, std_scaler_dae, data_input)
%#codegen

mean_output_dae = mean_scaler_dae';
std_output_dae = std_scaler_dae';

data_norm = (data_input - mean_output_dae)./std_output_dae;

== matlab function benchmark_ivan_PIANN/SO5_control_paper/Filter_Prediction/DAE_MLP1/Data Preprocessing Direct1/Denormalization Values ==
  data: mean_scaler_dae_out parameter; data_dir output; std_scaler_dae_out parameter; data_input input
function data_dir = descaler(mean_scaler_dae_out, std_scaler_dae_out, data_input)
%#codegen
data_dir = zeros(1, 48);

mean_output_3 = mean_scaler_dae_out';
std_output_3 = std_scaler_dae_out';

data_dir = std_output_3.*data_input + mean_output_3;

== matlab function benchmark_ivan_PIANN/SO5_control_paper/Filter_Prediction/DAE_MLP2/DAE/Predict RNN ==
  data: data_in input; prediction output; w_encoder_1 parameter; b_encoder_1 parameter; w_encoder_2 parameter; b_encoder_2 parameter; w_bottle parameter; b_bottle parameter; w_decoder_1 parameter; b_decoder_1 parameter; w_decoder_2 parameter; b_decoder_2 parameter; w_final parameter; b_final parameter
function prediction = predict_rnn(data_in, w_encoder_1, b_encoder_1, ...
    w_encoder_2, b_encoder_2, ...
    w_bottle, b_bottle, ...
    w_decoder_1, b_decoder_1, ...
    w_decoder_2, b_decoder_2, ...
    w_final, b_final)
%#codegen
    
    prediction = zeros(1,64);

    enc_1 = data_in*w_encoder_1 + b_encoder_1;
    enc_1(enc_1<0) = 0;
    enc_1_relu = enc_1;
    
    enc_2 = enc_1_relu*w_encoder_2 + b_encoder_2;
    enc_2(enc_2<0) = 0;
    enc_2_relu = enc_2;
    
    bottle = enc_2_relu*w_bottle + b_bottle;
    bottle(bottle<0) = 0;
    bottle_relu = bottle;
    
    dec_1 = bottle_relu*w_decoder_1 + b_decoder_1;
    dec_1(dec_1<0) = 0;
    dec_1_relu = dec_1;

    dec_2 = dec_1_relu*w_decoder_2 + b_decoder_2;
    dec_2(dec_2<0) = 0;
    dec_2_relu = dec_2;
    
    prediction = dec_2_relu*w_final + b_final;
end

== matlab function benchmark_ivan_PIANN/SO5_control_paper/Filter_Prediction/DAE_MLP2/Data Preprocesing Direct/Normalization Values ==
  data: mean_scaler_dae parameter; data_norm output; std_scaler_dae parameter; data_input input
function data_norm = scaler(mean_scaler_dae, std_scaler_dae, data_input)
%#codegen

mean_output_dae = mean_scaler_dae';
std_output_dae = std_scaler_dae';

data_norm = (data_input - mean_output_dae)./std_output_dae;
